simulink model "Joint_Position_Control"  (R2018b)
settings: Solver=ode4  StartTime=0.0  StopTime=10  FixedStep=0.005  RelTol=1e-3
settings Model: Creator=root  LastModifiedBy=root

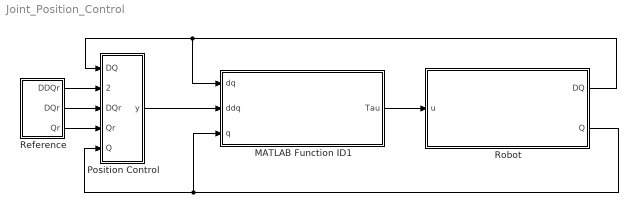
== system Joint_Position_Control ==
  MATLAB Function ID1 : MATLAB Function  TreatAsAtomicUnit=on
  Position Control : Subsystem
  Reference : Subsystem
  Robot : Subsystem
  wires:
  Position Control/1(y) -> MATLAB Function ID1/2(ddq)
  Robot/1(DQ) -> Position Control/1(DQ), MATLAB Function ID1/1(dq)
  Robot/2(Q) -> MATLAB Function ID1/3(q), Position Control/5(Q)
  Reference/2(DQr) -> Position Control/3(DQr)
  Reference/1(DDQr) -> Position Control/2(DDQr)
  Reference/3(Qr) -> Position Control/4(Qr)
  MATLAB Function ID1/1(Tau) -> Robot/1(u)

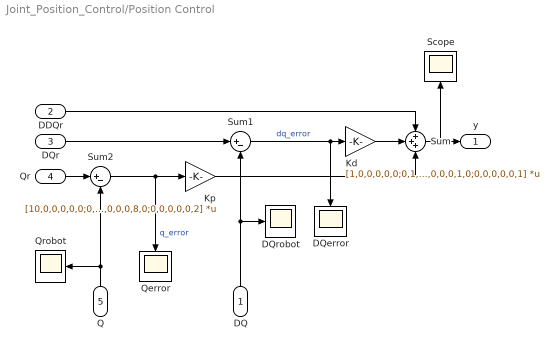
== system Joint_Position_Control/Position Control ==
  DQ : Inport
  DDQr : Inport  Port=2
  DQr : Inport  Port=3
  Qr : Inport  Port=4
  Q : Inport  Port=5
  DQerror : Scope
  DQrobot : Scope
  Kd : Gain  Gain=[1,0,0,0,0,0;0,1,0,0,0,0;0,0,1,0,0,0;0,0,0,1,0,0;0,0,0,0,1,0;0,0,0,0,0,1]  Multiplication=Matrix(K*u)
  Kp : Gain  Gain=[10,0,0,0,0,0;0,12,0,0,0,0;0,0,13,0,0,0;0,0,0,6,0,0;0,0,0,0,8,0;0,0,0,0,0,2]  Multiplication=Matrix(K*u)
  Qerror : Scope
  Qrobot : Scope
  Scope : Scope
  Sum : Sum  Inputs=+++
  Sum1 : Sum  Inputs=|+-
  Sum2 : Sum  Inputs=|+-
  y : Outport
  wires:
  Kd/1 -> Sum/2
  Kp/1 -> Sum/3
  Sum2/1 -> Qerror/1, Kp/1  "q_error"
  Qr/1 -> Sum2/1
  DQ/1 -> Sum1/2, DQrobot/1
  DQr/1 -> Sum1/1
  Sum/1 -> y/1, Scope/1
  Q/1 -> Qrobot/1, Sum2/2
  Sum1/1 -> Kd/1, DQerror/1  "dq_error"
  DDQr/1 -> Sum/1

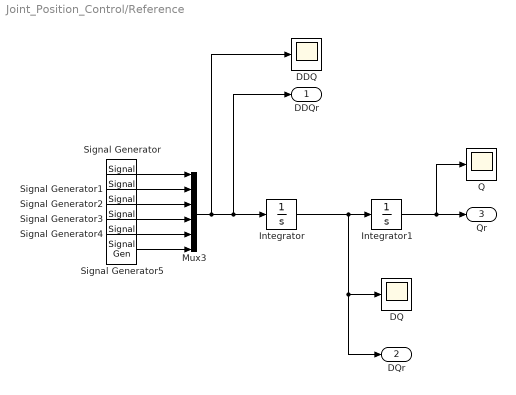
== system Joint_Position_Control/Reference ==
  DDQ : Scope
  DQ : Scope
  Integrator : Integrator
  Integrator1 : Integrator
  Mux3 : Mux  Inputs=6
  Q : Scope
  Signal Generator{,1..5} (6 alike) : SignalGenerator  WaveForm=square  Units=rad/sec
  DDQr : Outport
  DQr : Outport  Port=2
  Qr : Outport  Port=3
  wires:
  Signal Generator5/1 -> Mux3/6
  Signal Generator1/1 -> Mux3/2
  Signal Generator4/1 -> Mux3/5
  Signal Generator2/1 -> Mux3/3
  Signal Generator3/1 -> Mux3/4
  Signal Generator/1 -> Mux3/1
  Integrator/1 -> DQ/1, DQr/1, Integrator1/1
  Mux3/1 -> Integrator/1, DDQr/1, DDQ/1
  Integrator1/1 -> Q/1, Qr/1

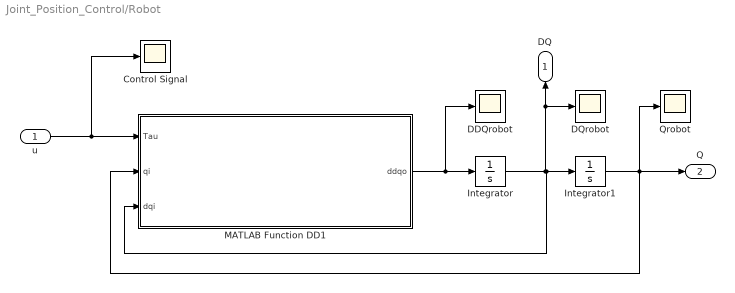
== system Joint_Position_Control/Robot ==
  u : Inport
  Control Signal : Scope
  DDQrobot : Scope
  DQrobot : Scope
  Integrator : Integrator  InitialCondition=[1,1,1,1,1,1]
  Integrator1 : Integrator  InitialCondition=[1,1,1,1,1,1]
  MATLAB Function DD1 : MATLAB Function  TreatAsAtomicUnit=on
  Qrobot : Scope
  DQ : Outport
  Q : Outport  Port=2
  wires:
  MATLAB Function DD1/1(ddqo) -> DDQrobot/1, Integrator/1
  Integrator/1 -> MATLAB Function DD1/3(dqi), Integrator1/1, DQrobot/1, DQ/1
  Integrator1/1 -> Qrobot/1, Q/1, MATLAB Function DD1/2(qi)
  u/1 -> Control Signal/1, MATLAB Function DD1/1(Tau)

== matlab function Joint_Position_Control/Robot/MATLAB Function DD1 ==
  data: Tau input; ddqo output; qi input; dqi input
function ddqo = DirectDynamics(Tau,qi,dqi)
    ddqo = zeros(6,1);
    coder.extrinsic('SolveSyms');
    c = zeros(6,1);
    m = zeros(6,6);
    g = zeros(6,1);
    [m,g,c] = SolveSyms(qi,dqi);
    ddqo = m\(Tau-c-g);
end

== matlab function Joint_Position_Control/MATLAB Function ID1 ==
  data: dq input; ddq input; q input; Tau output
function Tau   = Inverse_Dynamics(dq,ddq,q)
    Tau = zeros(6,1);
    c = zeros(6,1);
    m = zeros(6,6);
    g = zeros(6,1);
    coder.extrinsic('SolveSyms');
    [m,g,c] = SolveSyms(q,dq);
    Tau = (m*ddq + c + g);
end
